simulink model "part2model"  (R2019b)
settings: Solver=VariableStepAuto  StartTime=0.0  StopTime=4  RelTol=1e-3
values from neighbouring files (symbols this model uses):
  encGain = (2*pi)/4096    (= 0.00153398078789)    [DC_Motor_Analysis.m]    (also in Part2.m; Part3.m; lqrPoles.mat; robust.mat)
  K_fsf = place(A, B, [p p+.00001])    [Part2.m]
  kff = 1/dcGain_cl    [Part2.m]    (also in SS_lab.m = 0.0222222222222)
settings Model: Creator=justinf  LastModifiedBy=justinf
settings DebuggingCC: AlgebraicLoopMsg=none

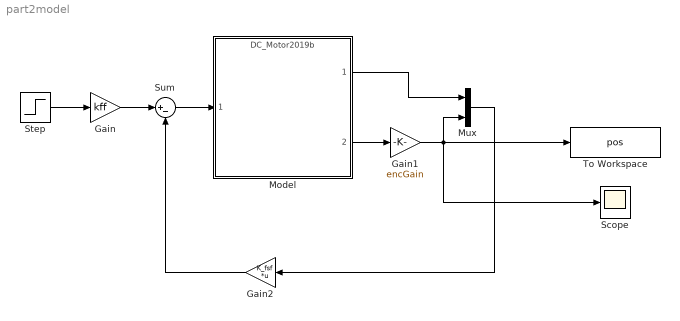
== system part2model ==
  Gain : Gain  Gain=kff
  Gain1 : Gain  Gain=encGain
  Gain2 : Gain  Gain=K_fsf  Multiplication=Matrix(K*u) (u vector)
  Model : ModelReference  ModelNameDialog=DC_Motor2019b.slxp  ModelReferenceVersion=1.20  CopyOfModelProtected=on
  Mux : Mux  Inputs=2
  Scope : Scope
  Step : Step  Time=0  SampleTime=0
  Sum : Sum  Inputs=|+-
  To Workspace : ToWorkspace  VariableName=pos  SampleTime=-1
  wires:
  Step/1 -> Gain/1
  Gain/1 -> Sum/1
  Sum/1 -> Model/1
  Model/2 -> Gain1/1
  Gain2/1 -> Sum/2
  Model/1 -> Mux/1
  Gain1/1 -> Scope/1, To Workspace/1, Mux/2
  Mux/1 -> Gain2/1
